simulink model "T2"  (R2015a)
settings: Solver=ode45  StartTime=0.0  StopTime=10.0  RelTol=1e-3
InitFcn:
  | Ra=1.3
  | m=0.13
  | kemf=0.7
  | La=0.001
  | l=0.2
values from neighbouring files (symbols this model uses):
  g = 9.81    [lqr_pendulo.m]    (also in pendulo.m)
undefined symbols (not defined in the file or in its folder): j, k
settings Model: Creator=Benjamin Nicolas  LastModifiedBy=Benjamin Nicolas

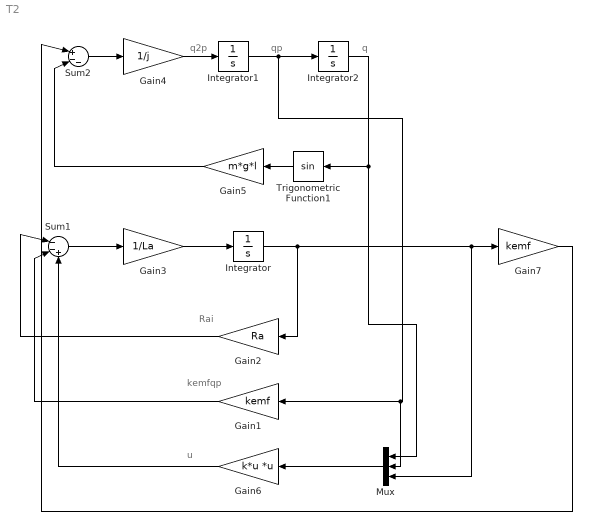
== system T2 ==
  note: u
  note: kemfqp
  note: Rai
  note: q
  note: qp
  note: q2p
  Gain1 : Gain  Gain=kemf
  Gain2 : Gain  Gain=Ra
  Gain3 : Gain  Gain=1/La
  Gain4 : Gain  Gain=1/j
  Gain5 : Gain  Gain=m*g*l
  Gain6 : Gain  Gain=k*u  Multiplication=Matrix(K*u) (u vector)
  Gain7 : Gain  Gain=kemf
  Integrator : Integrator
  Integrator1 : Integrator
  Integrator2 : Integrator
  Mux : Mux  Inputs=3
  Sum1 : Sum  Inputs=|--+
  Sum2 : Sum  Inputs=|+--
  Trigonometric Function1 : Trigonometry
  wires:
  Gain3/1 -> Integrator/1
  Mux/1 -> Gain6/1
  Sum1/1 -> Gain3/1
  Gain6/1 -> Sum1/3
  Gain1/1 -> Sum1/2
  Gain2/1 -> Sum1/1
  Trigonometric Function1/1 -> Gain5/1
  Gain5/1 -> Sum2/2
  Sum2/1 -> Gain4/1
  Gain4/1 -> Integrator1/1
  Integrator2/1 -> Mux/1, Trigonometric Function1/1
  Gain7/1 -> Sum2/1
  Integrator1/1 -> Mux/2, Gain1/1, Integrator2/1
  Integrator/1 -> Gain2/1, Mux/3, Gain7/1
